simulink model "ODE_T"  (R2019b)
settings: Solver=VariableStepAuto  StartTime=0.0  StopTime=10.0  RelTol=1e-3
settings Model: Creator=anna  LastModifiedBy=anna

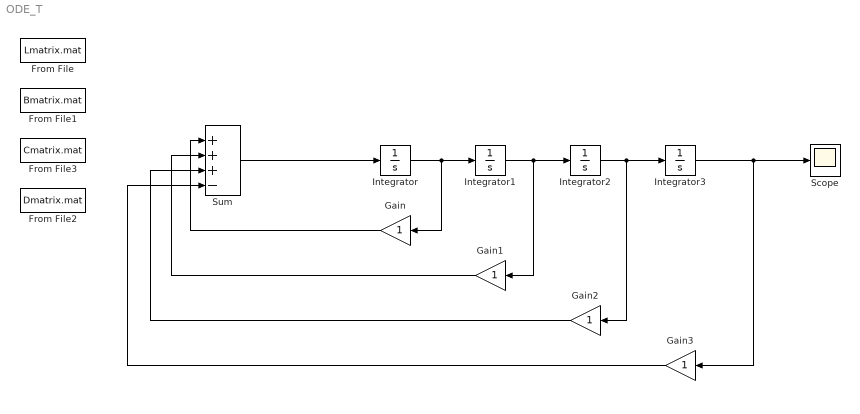
== system ODE_T ==
  From File : FromFile  FileName=Lmatrix.mat  SampleTime=0
  From File1 : FromFile  FileName=Bmatrix.mat  SampleTime=0
  From File2 : FromFile  FileName=Dmatrix.mat  SampleTime=0
  From File3 : FromFile  FileName=Cmatrix.mat  SampleTime=0
  Gain{,1..3} (4 alike) : Gain
  Integrator{,1..3} (4 alike) : Integrator
  Scope : Scope
  Sum : Sum  Inputs=|+++-
  wires:
  Integrator/1 -> Gain/1, Integrator1/1
  Sum/1 -> Integrator/1
  Integrator1/1 -> Gain1/1, Integrator2/1
  Integrator2/1 -> Gain2/1, Integrator3/1
  Integrator3/1 -> Gain3/1, Scope/1
  Gain/1 -> Sum/1
  Gain1/1 -> Sum/2
  Gain2/1 -> Sum/3
  Gain3/1 -> Sum/4
